simulink model "Demo_3D_Dynamics_cs"  (Simulink 7.6)
settings: Solver=ode5  SolverMode=SingleTasking  StartTime=0.0  StopTime=26  FixedStep=1/200  RelTol=1e-3
model workspace (MAT data in the model file):
  mbox_table.block_array(1).src = 'built-in/Subsystem'
  mbox_table.block_array(1).dest = 'Demo_3D_Dynamics_cs/BMW_X5_1'
  mbox_table.block_array(1).mode = 0
  mbox_table.block_array(2).src = 'simulink/Sinks/Out1'
  mbox_table.block_array(2).dest = 'Demo_3D_Dynamics_cs/BMW_X5_1/STATE_BMW_X5_1'
  mbox_table.block_array(2).mode = 0
  mbox_table.block_array(3).src = 'PreScanSimulinkLibrary/State'
  mbox_table.block_array(3).dest = 'Demo_3D_Dynamics_cs/STATE_BMW_X5_1'
  mbox_table.block_array(3).mode = 0
  mbox_table.block_array(4).src = 'PreScanSimulinkLibrary/PathFollower'
  mbox_table.block_array(4).dest = 'Demo_3D_Dynamics_cs/BMW_X5_1/PathFollower_1'
  mbox_table.block_array(4).mode = 0
  mbox_table.block_array(5).src = 'simulink/Sources/Constant'
  mbox_table.block_array(5).dest = 'Demo_3D_Dynamics_cs/BMW_X5_1/pos'
  mbox_table.block_array(5).mode = 0
  mbox_table.block_array(6).src = 'simulink/Sources/Constant'
  mbox_table.block_array(6).dest = 'Demo_3D_Dynamics_cs/BMW_X5_1/InitialVelocity'
  mbox_table.block_array(6).mode = 0
  mbox_table.block_array(7).src = 'PreScanSimulinkLibrary/Trajectories'
  mbox_table.block_array(7).dest = 'Demo_3D_Dynamics_cs/BMW_X5_1/Trajectories'
  mbox_table.block_array(7).mode = 0
  mbox_table.block_array(8).src = 'simulink/Sources/Constant'
  mbox_table.block_array(8).dest = 'Demo_3D_Dynamics_cs/BMW_X5_1/Trajectories/Trajectory_1_Offset'
  mbox_table.block_array(8).mode = 0
  mbox_table.block_array(9).src = 'PreScanSimulinkLibrary/Trajectory'
  mbox_table.block_array(9).dest = 'Demo_3D_Dynamics_cs/BMW_X5_1/Trajectories/Trajectory_1'
  mbox_table.block_array(9).mode = 0
  mbox_table.block_array(10).src = 'PreScanSimulinkLibrary/Traj2State'
  mbox_table.block_array(10).dest = 'Demo_3D_Dynamics_cs/BMW_X5_1/Trajectories/Traj2State1'
  mbox_table.block_array(10).mode = 0
  mbox_table.block_array(11).src = 'simulink/Sinks/Out1'
  mbox_table.block_array(11).dest = 'Demo_3D_Dynamics_cs/BMW_X5_1/Trajectories/State'
  mbox_table.block_array(11).mode = 0
  mbox_table.block_array(12).src = 'PreScanSimulinkLibrary/SELF'
  mbox_table.block_array(12).dest = 'Demo_3D_Dynamics_cs/SELF_BMW_X5_1'
  mbox_table.block_array(12).mode = 0
  mbox_table.block_array(13).src = 'simulink/Sources/In1'
  mbox_table.block_array(13).dest = 'Demo_3D_Dynamics_cs/BMW_X5_1/SELF_BMW_X5_1'
  mbox_table.block_array(13).mode = 0
  mbox_table.block_array(14).src = 'PreScanSimulinkLibrary/DemuxSELF'
  mbox_table.block_array(14).dest = 'Demo_3D_Dynamics_cs/BMW_X5_1/SELF_Demux'
  mbox_table.block_array(14).mode = 0
  mbox_table.block_array(15).src = 'simulink/Sinks/Out1'
  mbox_table.block_array(15).dest = 'Demo_3D_Dynamics_cs/BMW_X5_1/VISUWheels_BMW_X5_1'
  mbox_table.block_array(15).mode = 0
  mbox_table.block_array(16).src = 'PreScanSimulinkLibrary/VisuWheels'
  mbox_table.block_array(16).dest = 'Demo_3D_Dynamics_cs/VISUWheels_BMW_X5_1'
  mbox_table.block_array(16).mode = 0
  mbox_table.block_array(17).src = 'PreScanSimulinkLibrary/MuxWheels'
  mbox_table.block_array(17).dest = 'Demo_3D_Dynamics_cs/BMW_X5_1/VISUWheels_Mux'
  mbox_table.block_array(17).mode = 0
  mbox_table.block_array(18).src = 'PreScanSimulinkLibrary/Simple_Vehicle_Dynamics_3D'
  mbox_table.block_array(18).dest = 'Demo_3D_Dynamics_cs/BMW_X5_1/Dynamics_Simple_3D'
  mbox_table.block_array(18).mode = 0
  mbox_table.block_array(19).src = 'PreScanSimulinkLibrary/PreScan_Contact_Sensor'
  mbox_table.block_array(19).dest = 'Demo_3D_Dynamics_cs/BMW_X5_1/PreScan_Contact_Sensor'
  mbox_table.block_array(19).mode = 0
  mbox_table.block_array(20).src = 'SimCoreLibrary/SimCoreConfiguration'
  mbox_table.block_array(20).dest = 'Demo_3D_Dynamics_cs/SimCoreConfiguration'
  mbox_table.block_array(20).mode = 0
  mbox_table.block_array(21).src = 'SimCoreLibrary/Actuators'
  mbox_table.block_array(21).dest = 'Demo_3D_Dynamics_cs/Actuators'
  mbox_table.block_array(21).mode = 0
  mbox_table.block_array(22).src = 'SimCoreLibrary/SetActuators'
  mbox_table.block_array(22).dest = 'Demo_3D_Dynamics_cs/SetActuators'
  mbox_table.block_array(22).mode = 0
  mbox_table.block_array(23).src = 'SimCoreLibrary/GetSensors'
  mbox_table.block_array(23).dest = 'Demo_3D_Dynamics_cs/GetSensors'
  mbox_table.block_array(23).mode = 0
  mbox_table.block_array(24).src = 'SimCoreLibrary/SimCoreInfo'
  mbox_table.block_array(24).dest = 'Demo_3D_Dynamics_cs/SimCoreInfo'
  mbox_table.block_array(24).mode = 0
  mbox_table.block_array(25).src = 'PreScanSimulinkLibrary/Regenerate'
  mbox_table.block_array(25).dest = 'Demo_3D_Dynamics_cs/Regenerate'
  mbox_table.block_array(25).mode = 0
  mbox_table.block_array(26).src = 'PreScanSimulinkLibrary/Record for Replay  '
  mbox_table.block_array(26).dest = 'Demo_3D_Dynamics_cs/Record for Replay  '
  mbox_table.block_array(26).mode = 0
  mbox_table.block_array(27).src = 'PreScanSimulinkLibrary/Open Useful Blocks'
  mbox_table.block_array(27).dest = 'Demo_3D_Dynamics_cs/Open Useful Blocks'
  mbox_table.block_array(27).mode = 0
  mbox_table.block_array(28).src = 'PreScanSimulinkLibrary/PreScan Options   '
  mbox_table.block_array(28).dest = 'Demo_3D_Dynamics_cs/PreScan Options   '
  mbox_table.block_array(28).mode = 0
  mbox_table.block_array(29).src = 'built-in/Note'
  mbox_table.block_array(29).dest = 'Demo_3D_Dynamics_cs/Version:                  '
  mbox_table.block_array(29).mode = 0
  mbox_table.block_array(30).src = 'built-in/Note'
  mbox_table.block_array(30).dest = 'Demo_3D_Dynamics_cs/7.4.0'
  mbox_table.block_array(30).mode = 0
  mbox_table.block_array(31).src = 'built-in/Note'
  mbox_table.block_array(31).dest = 'Demo_3D_Dynamics_cs/Author(s):                '
  mbox_table.block_array(31).mode = 0
  mbox_table.block_array(32).src = 'built-in/Note'
  mbox_table.block_array(32).dest = 'Demo_3D_Dynamics_cs/N.A.'
  mbox_table.block_array(32).mode = 0
  mbox_table.block_array(33).src = 'built-in/Note'
  mbox_table.block_array(33).dest = 'Demo_3D_Dynamics_cs/Descriptive text:      '
  mbox_table.block_array(33).mode = 0
  mbox_table.block_array(34).src = 'built-in/Note'
  mbox_table.block_array(34).dest = 'Demo_3D_Dynamics_cs/N.A.'
  mbox_table.block_array(34).mode = 0
  mbox_table.block_array(35).src = 'built-in/Note'
  mbox_table.block_array(35).dest = 'Demo_3D_Dynamics_cs/ID
    | 
    | 18'
  mbox_table.block_array(35).mode = 0
  mbox_table.block_array(36).src = 'built-in/Note'
  mbox_table.block_array(36).dest = 'Demo_3D_Dynamics_cs/OBU-Beacon ID
    | 
    | '
  mbox_table.block_array(36).mode = 0
  mbox_table.block_array(37).src = 'built-in/Note'
  mbox_table.block_array(37).dest = 'Demo_3D_Dynamics_cs/TypeID
    | 
    | 1'
  mbox_table.block_array(37).mode = 0
  mbox_table.block_array(38).src = 'built-in/Note'
  mbox_table.block_array(38).dest = 'Demo_3D_Dynamics_cs/TypeTag
    | 
    | Car'
  mbox_table.block_array(38).mode = 0
  mbox_table.block_array(39).src = 'built-in/Note'
  mbox_table.block_array(39).dest = 'Demo_3D_Dynamics_cs/SD
    | 
    | Y'
  mbox_table.block_array(39).mode = 0
  mbox_table.block_array(40).src = 'built-in/Note'
  mbox_table.block_array(40).dest = 'Demo_3D_Dynamics_cs/CD
    | 
    | N'
  mbox_table.block_array(40).mode = 0
  mbox_table.block_array(41).src = 'built-in/Note'
  mbox_table.block_array(41).dest = 'Demo_3D_Dynamics_cs/Name
    | 
    | BMW_X5_1'
  mbox_table.block_array(41).mode = 0
  mbox_table.block_array(42).src = 'built-in/Note'
  mbox_table.block_array(42).dest = 'Demo_3D_Dynamics_cs/Num ID       OBU-Beacon ID     Type ID      Type Tag             SD        CD             Name                          '
  mbox_table.block_array(42).mode = 0
  mbox_table.block_array(43).src = 'built-in/Ground'
  mbox_table.block_array(43).dest = 'Demo_3D_Dynamics_cs/BMW_X5_1/Ground_1'
  mbox_table.block_array(43).mode = 1
  mbox_table.block_array(44).src = 'built-in/Ground'
  mbox_table.block_array(44).dest = 'Demo_3D_Dynamics_cs/BMW_X5_1/Ground_2'
  mbox_table.block_array(44).mode = 1
  mbox_table.block_array(45).src = 'built-in/Terminator'
  mbox_table.block_array(45).dest = 'Demo_3D_Dynamics_cs/BMW_X5_1/Terminator_1'
  mbox_table.block_array(45).mode = 1
  mbox_table.block_array(46).src = 'built-in/Ground'
  mbox_table.block_array(46).dest = 'Demo_3D_Dynamics_cs/BMW_X5_1/Ground_3'
  mbox_table.block_array(46).mode = 1
  mbox_table.block_array(47).src = 'built-in/Terminator'
  mbox_table.block_array(47).dest = 'Demo_3D_Dynamics_cs/BMW_X5_1/Terminator_2'
  mbox_table.block_array(47).mode = 1
  mbox_table.block_array(48).src = 'built-in/Terminator'
  mbox_table.block_array(48).dest = 'Demo_3D_Dynamics_cs/BMW_X5_1/Terminator_3'
  mbox_table.block_array(48).mode = 1
  mbox_table.block_array(49).src = 'built-in/Ground'
  mbox_table.block_array(49).dest = 'Demo_3D_Dynamics_cs/BMW_X5_1/Ground_4'
  mbox_table.block_array(49).mode = 1
  mbox_table.block_array(50).src = 'built-in/Terminator'
  mbox_table.block_array(50).dest = 'Demo_3D_Dynamics_cs/BMW_X5_1/Terminator_4'
  mbox_table.block_array(50).mode = 1
  mbox_table.block_array(51).src = 'built-in/Terminator'
  mbox_table.block_array(51).dest = 'Demo_3D_Dynamics_cs/BMW_X5_1/Terminator_5'
  mbox_table.block_array(51).mode = 1
  mbox_table.block_array(52).src = 'built-in/Terminator'
  mbox_table.block_array(52).dest = 'Demo_3D_Dynamics_cs/BMW_X5_1/Terminator_6'
  mbox_table.block_array(52).mode = 1
  mbox_table.block_array(53).src = 'built-in/Terminator'
  mbox_table.block_array(53).dest = 'Demo_3D_Dynamics_cs/BMW_X5_1/Terminator_7'
  mbox_table.block_array(53).mode = 1
  mbox_table.block_array(54).src = 'built-in/Terminator'
  mbox_table.block_array(54).dest = 'Demo_3D_Dynamics_cs/BMW_X5_1/Terminator_8'
  mbox_table.block_array(54).mode = 1
  mbox_table.block_array(55).src = 'built-in/Terminator'
  mbox_table.block_array(55).dest = 'Demo_3D_Dynamics_cs/BMW_X5_1/Terminator_9'
  mbox_table.block_array(55).mode = 1
  mbox_table.block_array(56).src = 'built-in/Terminator'
  mbox_table.block_array(56).dest = 'Demo_3D_Dynamics_cs/BMW_X5_1/Terminator_10'
  mbox_table.block_array(56).mode = 1
  mbox_table.block_array(57).src = 'built-in/Terminator'
  mbox_table.block_array(57).dest = 'Demo_3D_Dynamics_cs/BMW_X5_1/Terminator_11'
  mbox_table.block_array(57).mode = 1
  mbox_table.block_array(58).src = 'built-in/Terminator'
  mbox_table.block_array(58).dest = 'Demo_3D_Dynamics_cs/BMW_X5_1/Terminator_12'
  mbox_table.block_array(58).mode = 1
  mbox_table.block_array(59).src = 'built-in/Ground'
  mbox_table.block_array(59).dest = 'Demo_3D_Dynamics_cs/BMW_X5_1/Ground_5'
  mbox_table.block_array(59).mode = 1
  mbox_table.block_index : java.util.Hashtable (value not decoded)
  mbox_table.line_array(1).sys = 'Demo_3D_Dynamics_cs'
  mbox_table.line_array(1).line_id = 'L1'
  mbox_table.line_array(1).iport = 'STATE_BMW_X5_1/1'
  mbox_table.line_array(1).oport = 'BMW_X5_1/1'
  mbox_table.line_array(1).mode = 0
  mbox_table.line_array(2).sys = 'Demo_3D_Dynamics_cs/BMW_X5_1'
  mbox_table.line_array(2).line_id = 'L2'
  mbox_table.line_array(2).iport = 'PathFollower_1/1'
  mbox_table.line_array(2).oport = 'pos/1'
  mbox_table.line_array(2).mode = 0
  mbox_table.line_array(3).sys = 'Demo_3D_Dynamics_cs/BMW_X5_1'
  mbox_table.line_array(3).line_id = 'L3'
  mbox_table.line_array(3).iport = 'PathFollower_1/4'
  mbox_table.line_array(3).oport = 'InitialVelocity/1'
  mbox_table.line_array(3).mode = 0
  mbox_table.line_array(4).sys = 'Demo_3D_Dynamics_cs/BMW_X5_1/Trajectories'
  mbox_table.line_array(4).line_id = 'L4'
  mbox_table.line_array(4).iport = 'Traj2State1/1'
  mbox_table.line_array(4).oport = 'Trajectory_1/1'
  mbox_table.line_array(4).mode = 0
  mbox_table.line_array(5).sys = 'Demo_3D_Dynamics_cs/BMW_X5_1/Trajectories'
  mbox_table.line_array(5).line_id = 'L5'
  mbox_table.line_array(5).iport = 'Traj2State1/2'
  mbox_table.line_array(5).oport = 'Trajectory_1_Offset/1'
  mbox_table.line_array(5).mode = 0
  mbox_table.line_array(6).sys = 'Demo_3D_Dynamics_cs/BMW_X5_1/Trajectories'
  mbox_table.line_array(6).line_id = 'L6'
  mbox_table.line_array(6).iport = 'State/1'
  mbox_table.line_array(6).oport = 'Traj2State1/1'
  mbox_table.line_array(6).mode = 0
  mbox_table.line_array(7).sys = 'Demo_3D_Dynamics_cs'
  mbox_table.line_array(7).line_id = 'L7'
  mbox_table.line_array(7).iport = 'BMW_X5_1/1'
  mbox_table.line_array(7).oport = 'SELF_BMW_X5_1/1'
  mbox_table.line_array(7).mode = 0
  mbox_table.line_array(8).sys = 'Demo_3D_Dynamics_cs/BMW_X5_1'
  mbox_table.line_array(8).line_id = 'L8'
  mbox_table.line_array(8).iport = 'SELF_Demux/1'
  mbox_table.line_array(8).oport = 'SELF_BMW_X5_1/1'
  mbox_table.line_array(8).mode = 0
  mbox_table.line_array(9).sys = 'Demo_3D_Dynamics_cs/BMW_X5_1'
  mbox_table.line_array(9).line_id = 'L9'
  mbox_table.line_array(9).iport = 'VISUWheels_BMW_X5_1/1'
  mbox_table.line_array(9).oport = 'VISUWheels_Mux/1'
  mbox_table.line_array(9).mode = 0
  mbox_table.line_array(10).sys = 'Demo_3D_Dynamics_cs'
  mbox_table.line_array(10).line_id = 'L10'
  mbox_table.line_array(10).iport = 'VISUWheels_BMW_X5_1/1'
  mbox_table.line_array(10).oport = 'BMW_X5_1/2'
  mbox_table.line_array(10).mode = 0
  mbox_table.line_array(11).sys = 'Demo_3D_Dynamics_cs/BMW_X5_1'
  mbox_table.line_array(11).line_id = 'L11'
  mbox_table.line_array(11).iport = 'PreScan_Contact_Sensor/1'
  mbox_table.line_array(11).oport = 'Dynamics_Simple_3D/8'
  mbox_table.line_array(11).mode = 0
  mbox_table.line_array(12).sys = 'Demo_3D_Dynamics_cs/BMW_X5_1'
  mbox_table.line_array(12).line_id = 'L12'
  mbox_table.line_array(12).iport = 'Dynamics_Simple_3D/8'
  mbox_table.line_array(12).oport = 'PreScan_Contact_Sensor/1'
  mbox_table.line_array(12).mode = 0
  mbox_table.line_array(13).sys = 'Demo_3D_Dynamics_cs/BMW_X5_1'
  mbox_table.line_array(13).line_id = 'L13'
  mbox_table.line_array(13).iport = 'VISUWheels_Mux/3'
  mbox_table.line_array(13).oport = 'Dynamics_Simple_3D/2'
  mbox_table.line_array(13).mode = 0
  mbox_table.line_array(14).sys = 'Demo_3D_Dynamics_cs/BMW_X5_1'
  mbox_table.line_array(14).line_id = 'L14'
  mbox_table.line_array(14).iport = 'VISUWheels_Mux/4'
  mbox_table.line_array(14).oport = 'Dynamics_Simple_3D/4'
  mbox_table.line_array(14).mode = 0
  mbox_table.line_array(15).sys = 'Demo_3D_Dynamics_cs/BMW_X5_1'
  mbox_table.line_array(15).line_id = 'L15'
  mbox_table.line_array(15).iport = 'VISUWheels_Mux/5'
  mbox_table.line_array(15).oport = 'Dynamics_Simple_3D/5'
  mbox_table.line_array(15).mode = 0
  mbox_table.line_array(16).sys = 'Demo_3D_Dynamics_cs/BMW_X5_1'
  mbox_table.line_array(16).line_id = 'L16'
  mbox_table.line_array(16).iport = 'VISUWheels_Mux/6'
  mbox_table.line_array(16).oport = 'Dynamics_Simple_3D/6'
  mbox_table.line_array(16).mode = 0
  mbox_table.line_array(17).sys = 'Demo_3D_Dynamics_cs/BMW_X5_1'
  mbox_table.line_array(17).line_id = 'L17'
  mbox_table.line_array(17).iport = 'VISUWheels_Mux/7'
  mbox_table.line_array(17).oport = 'Dynamics_Simple_3D/7'
  mbox_table.line_array(17).mode = 0
  mbox_table.line_array(18).sys = 'Demo_3D_Dynamics_cs/BMW_X5_1'
  mbox_table.line_array(18).line_id = 'L18'
  mbox_table.line_array(18).iport = 'Dynamics_Simple_3D/1'
  mbox_table.line_array(18).oport = 'PathFollower_1/1'
  mbox_table.line_array(18).mode = 0
  mbox_table.line_array(19).sys = 'Demo_3D_Dynamics_cs/BMW_X5_1'
  mbox_table.line_array(19).line_id = 'L19'
  mbox_table.line_array(19).iport = 'Dynamics_Simple_3D/2'
  mbox_table.line_array(19).oport = 'PathFollower_1/2'
  mbox_table.line_array(19).mode = 0
  mbox_table.line_array(20).sys = 'Demo_3D_Dynamics_cs/BMW_X5_1'
  mbox_table.line_array(20).line_id = 'L20'
  mbox_table.line_array(20).iport = 'Dynamics_Simple_3D/3'
  mbox_table.line_array(20).oport = 'PathFollower_1/3'
  mbox_table.line_array(20).mode = 0
  mbox_table.line_array(21).sys = 'Demo_3D_Dynamics_cs/BMW_X5_1'
  mbox_table.line_array(21).line_id = 'L21'
  mbox_table.line_array(21).iport = 'Dynamics_Simple_3D/4'
  mbox_table.line_array(21).oport = 'PathFollower_1/4'
  mbox_table.line_array(21).mode = 0
  mbox_table.line_array(22).sys = 'Demo_3D_Dynamics_cs/BMW_X5_1'
  mbox_table.line_array(22).line_id = 'L22'
  mbox_table.line_array(22).iport = 'Dynamics_Simple_3D/6'
  mbox_table.line_array(22).oport = 'PathFollower_1/5'
  mbox_table.line_array(22).mode = 0
  mbox_table.line_array(23).sys = 'Demo_3D_Dynamics_cs/BMW_X5_1'
  mbox_table.line_array(23).line_id = 'L23'
  mbox_table.line_array(23).iport = 'PathFollower_1/6'
  mbox_table.line_array(23).oport = 'SELF_Demux/10'
  mbox_table.line_array(23).mode = 0
  mbox_table.line_array(24).sys = 'Demo_3D_Dynamics_cs/BMW_X5_1'
  mbox_table.line_array(24).line_id = 'L24'
  mbox_table.line_array(24).iport = 'STATE_BMW_X5_1/1'
  mbox_table.line_array(24).oport = 'Dynamics_Simple_3D/1'
  mbox_table.line_array(24).mode = 0
  mbox_table.line_array(25).sys = 'Demo_3D_Dynamics_cs/BMW_X5_1'
  mbox_table.line_array(25).line_id = 'l1'
  mbox_table.line_array(25).iport = 'Dynamics_Simple_3D/5'
  mbox_table.line_array(25).oport = 'Ground_1/1'
  mbox_table.line_array(25).mode = 1
  mbox_table.line_array(26).sys = 'Demo_3D_Dynamics_cs/BMW_X5_1'
  mbox_table.line_array(26).line_id = 'l2'
  mbox_table.line_array(26).iport = 'Dynamics_Simple_3D/7'
  mbox_table.line_array(26).oport = 'Ground_2/1'
  mbox_table.line_array(26).mode = 1
  mbox_table.line_array(27).sys = 'Demo_3D_Dynamics_cs/BMW_X5_1'
  mbox_table.line_array(27).line_id = 'l3'
  mbox_table.line_array(27).iport = 'Terminator_1/1'
  mbox_table.line_array(27).oport = 'Dynamics_Simple_3D/3'
  mbox_table.line_array(27).mode = 1
  mbox_table.line_array(28).sys = 'Demo_3D_Dynamics_cs/BMW_X5_1'
  mbox_table.line_array(28).line_id = 'l4'
  mbox_table.line_array(28).iport = 'PathFollower_1/2'
  mbox_table.line_array(28).oport = 'Ground_3/1'
  mbox_table.line_array(28).mode = 1
  mbox_table.line_array(29).sys = 'Demo_3D_Dynamics_cs/BMW_X5_1'
  mbox_table.line_array(29).line_id = 'l5'
  mbox_table.line_array(29).iport = 'Terminator_2/1'
  mbox_table.line_array(29).oport = 'PathFollower_1/6'
  mbox_table.line_array(29).mode = 1
  mbox_table.line_array(30).sys = 'Demo_3D_Dynamics_cs/BMW_X5_1'
  mbox_table.line_array(30).line_id = 'l6'
  mbox_table.line_array(30).iport = 'Terminator_3/1'
  mbox_table.line_array(30).oport = 'PathFollower_1/7'
  mbox_table.line_array(30).mode = 1
  mbox_table.line_array(31).sys = 'Demo_3D_Dynamics_cs/BMW_X5_1'
  mbox_table.line_array(31).line_id = 'l7'
  mbox_table.line_array(31).iport = 'PreScan_Contact_Sensor/3'
  mbox_table.line_array(31).oport = 'Ground_4/1'
  mbox_table.line_array(31).mode = 1
  mbox_table.line_array(32).sys = 'Demo_3D_Dynamics_cs/BMW_X5_1'
  mbox_table.line_array(32).line_id = 'l8'
  mbox_table.line_array(32).iport = 'Terminator_4/1'
  mbox_table.line_array(32).oport = 'SELF_Demux/3'
  mbox_table.line_array(32).mode = 1
  mbox_table.line_array(33).sys = 'Demo_3D_Dynamics_cs/BMW_X5_1'
  mbox_table.line_array(33).line_id = 'l9'
  mbox_table.line_array(33).iport = 'Terminator_5/1'
  mbox_table.line_array(33).oport = 'SELF_Demux/4'
  mbox_table.line_array(33).mode = 1
  mbox_table.line_array(34).sys = 'Demo_3D_Dynamics_cs/BMW_X5_1'
  mbox_table.line_array(34).line_id = 'l10'
  mbox_table.line_array(34).iport = 'Terminator_6/1'
  mbox_table.line_array(34).oport = 'SELF_Demux/5'
  mbox_table.line_array(34).mode = 1
  mbox_table.line_array(35).sys = 'Demo_3D_Dynamics_cs/BMW_X5_1'
  mbox_table.line_array(35).line_id = 'l11'
  mbox_table.line_array(35).iport = 'Terminator_7/1'
  mbox_table.line_array(35).oport = 'SELF_Demux/7'
  mbox_table.line_array(35).mode = 1
  mbox_table.line_array(36).sys = 'Demo_3D_Dynamics_cs/BMW_X5_1'
  mbox_table.line_array(36).line_id = 'l12'
  mbox_table.line_array(36).iport = 'Terminator_8/1'
  mbox_table.line_array(36).oport = 'SELF_Demux/8'
  mbox_table.line_array(36).mode = 1
  mbox_table.line_array(37).sys = 'Demo_3D_Dynamics_cs/BMW_X5_1'
  mbox_table.line_array(37).line_id = 'l13'
  mbox_table.line_array(37).iport = 'Terminator_9/1'
  mbox_table.line_array(37).oport = 'SELF_Demux/9'
  mbox_table.line_array(37).mode = 1
  mbox_table.line_array(38).sys = 'Demo_3D_Dynamics_cs/BMW_X5_1'
  mbox_table.line_array(38).line_id = 'l14'
  mbox_table.line_array(38).iport = 'Terminator_10/1'
  mbox_table.line_array(38).oport = 'SELF_Demux/11'
  mbox_table.line_array(38).mode = 1
  mbox_table.line_array(39).sys = 'Demo_3D_Dynamics_cs/BMW_X5_1'
  mbox_table.line_array(39).line_id = 'l15'
  mbox_table.line_array(39).iport = 'Terminator_11/1'
  mbox_table.line_array(39).oport = 'SELF_Demux/12'
  mbox_table.line_array(39).mode = 1
  mbox_table.line_array(40).sys = 'Demo_3D_Dynamics_cs/BMW_X5_1'
  mbox_table.line_array(40).line_id = 'l16'
  mbox_table.line_array(40).iport = 'Terminator_12/1'
  mbox_table.line_array(40).oport = 'Trajectories/1'
  mbox_table.line_array(40).mode = 1
  mbox_table.line_array(41).sys = 'Demo_3D_Dynamics_cs/BMW_X5_1'
  mbox_table.line_array(41).line_id = 'l17'
  mbox_table.line_array(41).iport = 'VISUWheels_Mux/2'
  mbox_table.line_array(41).oport = 'Ground_5/1'
  mbox_table.line_array(41).mode = 1
  mbox_table.line_index : java.util.Hashtable (value not decoded)
  mbox_table.next_linenr = 25
  mbox_table.next_termlinenr = 18
  model_closed = 0
  sim_status = 0
PreLoadFcn:
  | check_NUTS_defined;
  | 
  | assignin('base',['model_closed_' bdroot],false);
InitFcn:
  | PreScanExperimentInitFcn(bdroot)
StopFcn:
  | PreScanExperimentStopFcn(bdroot)
undefined symbols (not defined in the file): DiscIntNeverNeededParam, x_ini_VRML, y_ini_VRML, z_ini_VRML
libraries: simulink x37, simulink_extras x11, PreScanSimulinkLibrary x10, simulink_need_slupdate x1, PreScanUsefulBlocks x1
(part 1 of 5)
CloseFcn:
  | evalin('base',['clear model_closed_' bdroot]);
settings Model: Creator=PRESCAN  LastModifiedBy=buildbot
settings OptimizationCC: InitFltsAndDblsToZero=on
settings DebuggingCC: SaveWithParameterizedLinksMsg=none  SignalResolutionControl=TryResolveAllWithWarning  SolverPrmCheckMsg=none  MultiTaskDSMMsg=warning  MultiTaskCondExecSysMsg=none
settings RTWCC: IncludeERTFirstTime=on
settings GRTTargetCC: TargetFcnLib=ansi_tfl_tmw.mat

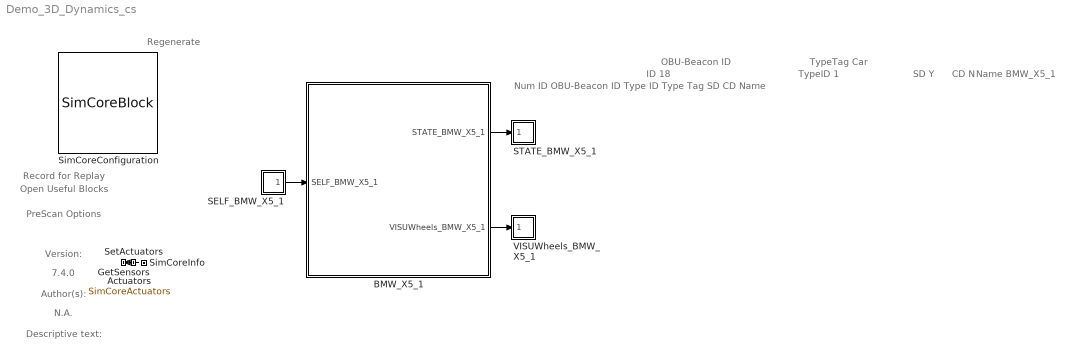
== system Demo_3D_Dynamics_cs ==
  note: Regenerate
  note: Record for Replay
  note: Open Useful Blocks
  note: PreScan Options
  note: Version:
  note: 7.4.0
  note: Author(s):
  note: N.A.
  note: Descriptive text:
  note: ID
      |
      | 18
  note: OBU-Beacon ID
  note: TypeID
      |
      | 1
  note: TypeTag
      |
      | Car
  note: SD
      |
      | Y
  note: CD
      |
      | N
  note: Name
      |
      | BMW_X5_1
  note: Num ID OBU-Beacon ID Type ID Type Tag SD CD Name
  Actuators : DataStoreMemory  Tag=Actuators  DataStoreName=SimCoreActuators  InitialValue=zeros(43,1)
      settings: DeleteFcn=PreScanBlockDeleteFcn;
  BMW_X5_1 : Subsystem  Tag=WorldObjectSubSystem  InitFcn=UniqueId = '276';
      mask Display: image(imread('BMW_X5.jpg'));color('white');text(0,0,' ID=18\n')
  GetSensors : Subsystem  Tag=GetSensors  Priority=2  mask(PreScan Simulation Core Block){NrOfSensors=8, TimeStep=10/200}
      mask prompts: NrOfSensors "Number of sensor values"; TimeStep "Timestep [s]"
      mask help:
      | Please do not remove this block from the PreScan compilation sheet,
      | as it contains essential configuration parameters for a PreScan simulation.
      settings: DeleteFcn=PreScanBlockDeleteFcn;
  SELF_BMW_X5_1 : Subsystem  Tag=SELF  Priority=3  mask(PreScan Source Block: SELF){PortName=SELF_BMW_X5_1, PortIndex=0, PortWidth=8, TimeStep=10/200}
      mask prompts: PortName "Auto-Assigned: Port Name [-]"; PortIndex "Auto-Assigned: Port Index [-]"; PortWidth "Auto-Assigned: Port Dimensions"; TimeStep "Auto-Assigned: Upload Period [s]"
      mask help:
      | The SELF port shows (state) information of the actor itself. The outputs are position in the experiment's axis system and the GPS coordinates, and the object's absolute velocity and compass heading.
      |
      | For more information, please click Help.
      settings: DeleteFcn=PreScanBlockDeleteFcn;
      mask Help: eval('openHelp(462)')
      mask Display: image(imread('GPS.png'))
  STATE_BMW_X5_1 : Subsystem  Tag=State  Priority=0  mask(PreScan Sink Block: State){x0=40, y0=28.25, z0=0.69, Roll0=0, Pitch0=0, Yaw0=0, TimeStep=10/200}
      mask prompts: x0 "Ini x-position VEHICLE wrt GLOBAL axis system [m]"; y0 "Ini y-position VEHICLE wrt GLOBAL axis system [m]"; z0 "Ini z-position VEHICLE wrt GLOBAL axis system [m]"; Roll0 "Ini roll-angle BODY wrt VEHICLE axis system [deg]"; Pitch0 "Ini pitch-angle BODY wrt VEHICLE axis system [deg]"; Yaw0 "Ini yaw-angle VEHICLE wrt GLOBAL axis system [deg]"; TimeStep "Time Step [s]"
      mask help:
      | The Actor State contains a vector signal of size (9x1), containing the following signals:
      |
      | -  Position                  (x,y,z)                                     [m]
      | -  Velocity                  (vx,vy,vz)                               [m/s]
      | -  Angles                    (Roll, Pitch, Yaw)                   [rad]
      |
      | The Actor state is defined in the global axis system.
      | The state is superponed on the Initial position defined in the GUI.
      |
      | For more information, please click Help.
      settings: DeleteFcn=PreScanBlockDeleteFcn;
      mask Help: eval('openHelp(222)')
      mask Display: image(imread('State.png'))
  SetActuators : Subsystem  Tag=SetActuators  Priority=1  mask(PreScan Simulation Core Block){TimeStep=10/200, NrOfActuators=43}
      mask prompts: TimeStep "Timestep [s]"; NrOfActuators "Number of actuator values"
      mask help:
      | Please do not remove this block from the PreScan compilation sheet,
      | as it contains essential configuration parameters for a PreScan simulation.
      settings: DeleteFcn=PreScanBlockDeleteFcn;
  SimCoreConfiguration : M-S-Function  Tag=SimCoreConfiguration  Description=2F8DE11AFA9E2D1E60DFF0BB6A25510BB705AF952DBBD0EADC2C0AF755B6A15B  FunctionName=SimCoreBlock  Parameters=ExperimentXML PortsXML SimulationCore HostName CheckStart EnableLog RfR EnableGPUAccel ShowComputationTime  mask(PreScan Simulation Core Configurator){SimulationCore=NUTS, HostName=0, CheckStart=0, prescanversion='7.4.0', EnableLog=off, RfR=0, EnableGPUAccel=off, ShowComputationTime=off}
      mask prompts: SimulationCore "Simulation Core"; HostName "Simulation Host"; CheckStart "Show START Dialog"; prescanversion "PreScan Version"; EnableLog "Create TA Log"; RfR "Record for Replay"; EnableGPUAccel "Enable GPU Acceleration"; ShowComputationTime "Show ComputationTime Scope"
      mask help:
      | Please do not remove this block from the PreScan compilation sheet,
      | as it contains essential configuration parameter for a PreScan simulation.
      mask init:
      | model = bdroot;
      | ExperimentXML = [model(1:end-3) '.pex'];
      | PortsXML = [model '_ports.pcd'];
      settings: DeleteFcn=PreScanBlockDeleteFcn;  ModelCloseFcn=assignin('base',['model_closed_' bdroot],true);
      mask Help: eval('openHelp(812)')
      mask Display: image(imread('prescanlogo.ico'))
  SimCoreInfo : Subsystem  Tag=SimCoreInfo
  VISUWheels_BMW_X5_1 : Subsystem  Tag=VisuWheels  Priority=0
      settings: DeleteFcn=PreScanBlockDeleteFcn;
      mask Type: PreScan Sink Block: VisuWheels
      mask Description:
      | The VisuWheels block provides a way to animate the wheels of a vehicle, with steering, rotation (because of velocity) and z-displacement.
      | 
      | For more information, please click Help.
      mask Help: eval('openHelp(223)')
      mask Display: image(imread('wheel.png'))
  wires:
  BMW_X5_1/1(STATE_BMW_X5_1) -> STATE_BMW_X5_1/1(State)
  SELF_BMW_X5_1/1(U) -> BMW_X5_1/1(SELF_BMW_X5_1)
  BMW_X5_1/2(VISUWheels_BMW_X5_1) -> VISUWheels_BMW_X5_1/1(Wheels)
  SetActuators/1(dummy) -> GetSensors/1(dummy)

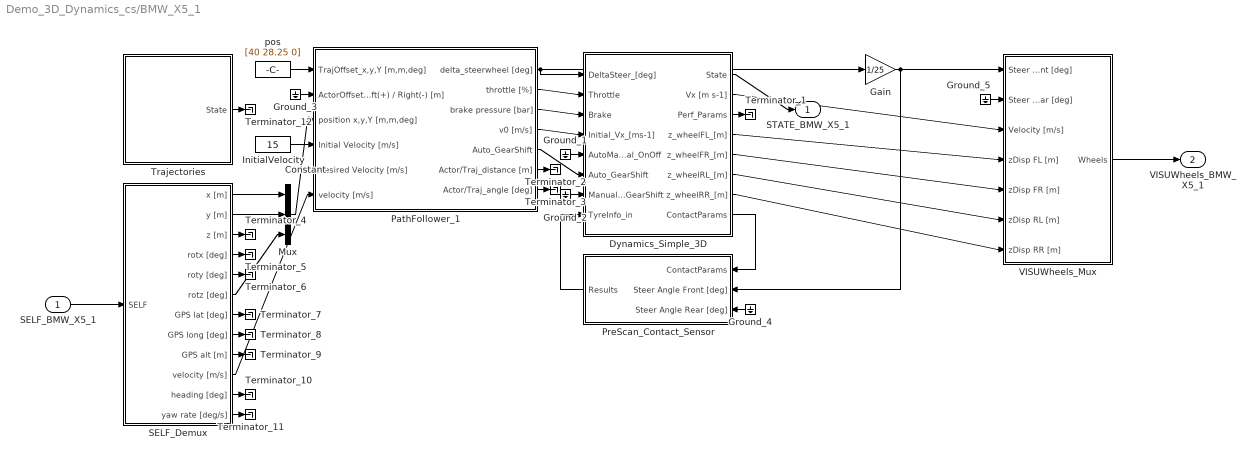
== system Demo_3D_Dynamics_cs/BMW_X5_1 ==
  SELF_BMW_X5_1 : Inport  Tag=SELFInport
  Constant : Constant  Value=15
  Dynamics_Simple_3D : Subsystem  Tag=Simple_Vehicle_Dynamics_3D  mask(PreScan Block: Simple Dynamics 3D){Migrate=on, TimeStep=1/200, ComputationMode=Continuous_Time}
      mask prompts: Migrate "Migrate. During migration this block will be replaced by a newer one."; TimeStep "Auto assigned: Time Step [s]"; ComputationMode "Computation mode:"
      mask help:
      | The Simple Dynamics Model is selected in the GUI to simulate vehicle dynamics behavior.
      |
      | The Simple Dynamics Model is completely open to the user. The parameters of this model can be set in the Simple Dynamics dialog in the GUI.
      |
      | For more information, please click Help.
      mask init:
      | p = SimpleDyn_pars;
      settings: DeleteFcn=PreScanBlockDeleteFcn;
      mask Help: eval('openHelp(234)')
      mask Display:
      | image(imread('SimpleDyn.png'))
      | port_label('input', 1, '{\delta}_S_t_ _e_e_r [deg]','texmode','on')
      | port_label('input', 2, 'Throttle [%]')
      | port_label('input', 3, 'Brake Pres [bar]')
      | port_label('input', 4, 'V_0 [ms-1]','texmode','on')
      | port_label('input', 5, 'Auto=[0]/Manual=[1]')
      | port_label('input', 6, 'Auto_GearShift')
      | port_label('input', 7, 'Manual_GearShift')
      | port_label('input', 8, 'TyreInfo_in')
      | port_label('output', 1, 'State')
      | port_label('output', 2, 'Vx [ms-1]')
      | port_label('output', 3, 'Perf Params')
      | port_label('output', 4, 'zDispFL[m]')
      | port_label('output', 5, 'zDispFR[m]')
      | port_label('output', 6, 'zDispRL[m]')
      | port_label('output', 7, 'zDispRR[m]')
  Gain : Gain  Gain=1/25
  Ground_{1..5} (5 alike) : Ground
  InitialVelocity : Constant  Tag=InitialVelocity  Value=15
  Mux : Mux  Inputs=3
  PathFollower_1 : Subsystem  Tag=pathFollower  mask(PreScan Block: Path Follower){Migrate=on, FileName='Trajectory_1.mat', TunableSteeringGain=1, XShifting_wrt_COG=0}
      mask prompts: Migrate "Migrate. During migration this block will be replaced by a newer one."; FileName "Trajectory Name"; TunableSteeringGain "TunableSteeringGain [-]"; XShifting_wrt_COG "XShifting_wrt_COG [m]"
      mask help:
      | The Path Follower Model is selected in the GUI to simulate driver behavior.
      |
      | For more information, please click Help.
      mask init:
      | load(['trajectories/',eval(FileName)])
      | traject=trajectory';
      | 
      | Traj_x=traject(:,2);
      | Traj_y=traject(:,3);
      | Traj_z=traject(:,4);
      | Traj_vx=traject(:,8);
      | Traj_vy=traject(:,9);
      | Traj_vz=traject(:,10);
      mask Help: eval('openHelp(232)')
  PreScan_Contact_Sensor : Subsystem  Tag=PreScan_Contact_Sensor  mask(PreScan Block: PreScan Contact Sensor){x0=40, y0=28.25, z0=0.69, Roll0=0, Pitch0=0, Yaw0=0, wheelRadius=0.37, hcog=0.69, b=1.69, TimeStep=1/200}
      mask prompts: x0 "Ini x-position VEHICLE wrt GLOBAL axis system [m]"; y0 "Ini y-position VEHICLE wrt GLOBAL axis system [m]"; z0 "Ini z-position VEHICLE wrt GLOBAL axis system [m]"; Roll0 "Ini roll-angle BODY wrt VEHICLE axis system [deg]"; Pitch0 "Ini pitch-angle BODY wrt VEHICLE axis system [deg]"; Yaw0 "Ini yaw-angle VEHICLE wrt GLOBAL axis system [deg]"; wheelRadius "Wheel Radius [m]"; hcog "Dynamics: hCoG [m]"; b "Dynamics: b [m]"; TimeStep "Time Step [s]"
      mask help:
      | This block encapsulates the base Contact sensor.
      |
      | It takes input parameters from the PreScan 3D vehicle dynamics block and outputs contact results.
      mask Help: eval('openHelp(251)')
  SELF_Demux : Subsystem  Tag=DemuxSELF
      settings: DeleteFcn=PreScanBlockDeleteFcn;
      mask Type: PreScan Demux Block:
      mask Display:
      | port_label('output',1,'x [m]')
      | port_label('output',2,'y [m]')
      | port_label('output',3,'z [m]','texmode','on')
      | port_label('output',4,'Rotx [deg]','texmode','on')
      | port_label('output',5,'Roty [deg]','texmode','on')
      | port_label('output',6,'Rotz [deg]','texmode','on')
      | port_label('output',7,'GPS lat [deg]','texmode','on')
      | port_label('output',8,'GPS long [deg]','texmode','on')
      | port_label('output',9,'GPS alt [m]','texmode','on')
      | port_label('output',10,'Velocity [m/s]')
      | port_label('output',11,'Heading [deg]')
      | port_label('output',12,'Yaw rate [deg/s]')
  Terminator_{1..12} (12 alike) : Terminator
  Trajectories : Subsystem  Tag=Trajectories
      settings: DeleteFcn=PreScanBlockDeleteFcn;
      mask Type: PreScan Source Block: Trajectories
      mask Description:
      | The Trajectory block contains the trajectories defined in the PreScan Experiment Editor. The output of the trajectory block is the (vehicle) State.
      | 
      | For more information, please click Help.
      mask Help: eval('openHelp(312)')
      mask Display: image(imread('Trajectory.png'));
  VISUWheels_Mux : Subsystem  Tag=MuxWheels  mask(PreScan Mux Block:){TimeStep=10/200}
      mask prompts: TimeStep "Auto Assigned: Time Step [s]"
      settings: DeleteFcn=PreScanBlockDeleteFcn;
  pos : Constant  Tag=pos  Value=[40 28.25 0]
  STATE_BMW_X5_1 : Outport  Tag=StateOutport
  VISUWheels_BMW_X5_1 : Outport  Tag=VisuWheelsOutport  Port=2  SampleTime=10/200
  wires:
  pos/1 -> PathFollower_1/1(TrajOffset_x,y,Y [m,m,deg])
  InitialVelocity/1 -> PathFollower_1/4(Initial Velocity [m/s])
  SELF_BMW_X5_1/1 -> SELF_Demux/1(SELF)
  VISUWheels_Mux/1(Wheels) -> VISUWheels_BMW_X5_1/1
  Dynamics_Simple_3D/8(ContactParams) -> PreScan_Contact_Sensor/1(ContactParams)
  PreScan_Contact_Sensor/1(Results) -> Dynamics_Simple_3D/8(TyreInfo_in)
  Dynamics_Simple_3D/2(Vx [m s-1]) -> VISUWheels_Mux/3(Velocity [m/s])
  Dynamics_Simple_3D/4(z_wheelFL_[m]) -> VISUWheels_Mux/4(zDisp FL [m])
  Dynamics_Simple_3D/5(z_wheelFR_[m]) -> VISUWheels_Mux/5(zDisp FR [m])
  Dynamics_Simple_3D/6(z_wheelRL_[m]) -> VISUWheels_Mux/6(zDisp RL [m])
  Dynamics_Simple_3D/7(z_wheelRR_[m]) -> VISUWheels_Mux/7(zDisp RR [m])
  PathFollower_1/1(delta_steerwheel [deg]) -> Dynamics_Simple_3D/1(DeltaSteer_[deg]), Gain/1
  PathFollower_1/2(throttle [%]) -> Dynamics_Simple_3D/2(Throttle)
  PathFollower_1/3(brake pressure [bar]) -> Dynamics_Simple_3D/3(Brake)
  PathFollower_1/4(v0 [m/s]) -> Dynamics_Simple_3D/4(Initial_Vx_[ms-1])
  PathFollower_1/5(Auto_GearShift) -> Dynamics_Simple_3D/6(Auto_GearShift)
  Dynamics_Simple_3D/1(State) -> STATE_BMW_X5_1/1
  Gain/1 -> VISUWheels_Mux/1(Steer Angle Front [deg]), PreScan_Contact_Sensor/2(Steer Angle Front [deg])
  SELF_Demux/10(velocity [m/s]) -> PathFollower_1/6(velocity [m/s])
  Mux/1 -> PathFollower_1/3(position x,y,Y [m,m,deg])
  SELF_Demux/6(rotz [deg]) -> Mux/3
  Constant/1 -> PathFollower_1/5(Desired Velocity [m/s])
  SELF_Demux/2(y [m]) -> Mux/2
  SELF_Demux/1(x [m]) -> Mux/1
  Ground_1/1 -> Dynamics_Simple_3D/5(AutoManual_OnOff)
  Ground_2/1 -> Dynamics_Simple_3D/7(Manual_GearShift)
  Dynamics_Simple_3D/3(Perf_Params) -> Terminator_1/1
  Ground_3/1 -> PathFollower_1/2(ActorOffset_Left(+) / Right(-) [m])
  PathFollower_1/6(Actor/Traj_distance [m]) -> Terminator_2/1
  PathFollower_1/7(Actor/Traj_angle [deg]) -> Terminator_3/1
  Ground_4/1 -> PreScan_Contact_Sensor/3(Steer Angle Rear [deg])
  SELF_Demux/3(z [m]) -> Terminator_4/1
  SELF_Demux/4(rotx [deg]) -> Terminator_5/1
  SELF_Demux/5(roty [deg]) -> Terminator_6/1
  SELF_Demux/7(GPS lat [deg]) -> Terminator_7/1
  SELF_Demux/8(GPS long [deg]) -> Terminator_8/1
  SELF_Demux/9(GPS alt [m]) -> Terminator_9/1
  SELF_Demux/11(heading [deg]) -> Terminator_10/1
  SELF_Demux/12(yaw rate [deg/s]) -> Terminator_11/1
  Trajectories/1(State) -> Terminator_12/1
  Ground_5/1 -> VISUWheels_Mux/2(Steer Angle Rear [deg])

== system Demo_3D_Dynamics_cs/GetSensors ==
  dummy : Inport
  GetSensors : M-S-Function  FunctionName=GetSensorsBlock  Parameters=TimeStep NrOfSensors
  tag scope: SimCoreSensors=global
  wires:
  GetSensors/1 -> [SimCoreSensors]
  dummy/1 -> GetSensors/1

== system Demo_3D_Dynamics_cs/SELF_BMW_X5_1 ==
  Selector : Selector  IndexMode=Zero-based  IndexOptions=Starting index (dialog)  Indices=PortIndex  OutputSizes=PortWidth(1)
  U : Outport
  wires:
  Selector/1 -> U/1
  [SimCoreSensors] -> Selector/1

== system Demo_3D_Dynamics_cs/STATE_BMW_X5_1 ==
  State : Inport  SampleTime=TimeStep
  Acceleration : Subsystem  mask(ToSensorWorld){PortName=Acceleration_BMW_X5_1, PortIndex=6, PortWidth=3, TimeStep=10/200}
      mask prompts: PortName "Port Name [-]"; PortIndex "Index [-]"; PortWidth "Port Dimensions [-]"; TimeStep "Upload Period [s]"
      mask help: Sends signal(s) from Simulink to the Sensor World
      mask Help:
      | Sends signal(s) from Simulink to the Sensor World.
      | 
      | - Port Name [-]: specifies the name of the output terminal of the Simulink block.
      | - Index [-]: specifies the start position in the output vector sent to the Sensor World
      | - Port dimensions [-]: specifies the width (number of scalars) of the output port
      | - Upload period [s]: specifies the upload period (in seconds) of the port.
      mask Display: port_label('input', 1, PortName)
  Demux : Demux  Outputs=5
  Position : Subsystem  mask(ToSensorWorld){PortName=Position_BMW_X5_1, PortIndex=0, PortWidth=3, TimeStep=10/200}
      mask prompts: PortName "Port Name [-]"; PortIndex "Index [-]"; PortWidth "Port Dimensions [-]"; TimeStep "Upload Period [s]"
      mask help: Sends signal(s) from Simulink to the Sensor World
      mask Help:
      | Sends signal(s) from Simulink to the Sensor World.
      | 
      | - Port Name [-]: specifies the name of the output terminal of the Simulink block.
      | - Index [-]: specifies the start position in the output vector sent to the Sensor World
      | - Port dimensions [-]: specifies the width (number of scalars) of the output port
      | - Upload period [s]: specifies the upload period (in seconds) of the port.
      mask Display: port_label('input', 1, PortName)
  RPY : Subsystem  mask(ToSensorWorld){PortName=RPY_BMW_X5_1, PortIndex=9, PortWidth=3, TimeStep=10/200}
      mask prompts: PortName "Port Name [-]"; PortIndex "Index [-]"; PortWidth "Port Dimensions [-]"; TimeStep "Upload Period [s]"
      mask help: Sends signal(s) from Simulink to the Sensor World
      mask Help:
      | Sends signal(s) from Simulink to the Sensor World.
      | 
      | - Port Name [-]: specifies the name of the output terminal of the Simulink block.
      | - Index [-]: specifies the start position in the output vector sent to the Sensor World
      | - Port dimensions [-]: specifies the width (number of scalars) of the output port
      | - Upload period [s]: specifies the upload period (in seconds) of the port.
      mask Display: port_label('input', 1, PortName)
  Velocity : Subsystem  mask(ToSensorWorld){PortName=Velocity_BMW_X5_1, PortIndex=3, PortWidth=3, TimeStep=10/200}
      mask prompts: PortName "Port Name [-]"; PortIndex "Index [-]"; PortWidth "Port Dimensions [-]"; TimeStep "Upload Period [s]"
      mask help: Sends signal(s) from Simulink to the Sensor World
      mask Help:
      | Sends signal(s) from Simulink to the Sensor World.
      | 
      | - Port Name [-]: specifies the name of the output terminal of the Simulink block.
      | - Index [-]: specifies the start position in the output vector sent to the Sensor World
      | - Port dimensions [-]: specifies the width (number of scalars) of the output port
      | - Upload period [s]: specifies the upload period (in seconds) of the port.
      mask Display: port_label('input', 1, PortName)
  iniBODYAngles wrtVEH [rad] : Constant  Value=[Roll0 Pitch0 0]  SampleTime=TimeStep
  iniVEHAngles wrtGLOB [rad] : Constant  Value=[0 0 Yaw0]  SampleTime=TimeStep
  iniVEHposition wrtGLOB [m] : Constant  Value=[x0 y0 z0]  SampleTime=TimeStep
  state2FullState : PreScanSimulinkLibrary/state2FullState  SystemSampleTime=-1
  velRPY : Subsystem  mask(ToSensorWorld){PortName=velRPY_BMW_X5_1, PortIndex=12, PortWidth=3, TimeStep=10/200}
      mask prompts: PortName "Port Name [-]"; PortIndex "Index [-]"; PortWidth "Port Dimensions [-]"; TimeStep "Upload Period [s]"
      mask help: Sends signal(s) from Simulink to the Sensor World
      mask Help:
      | Sends signal(s) from Simulink to the Sensor World.
      | 
      | - Port Name [-]: specifies the name of the output terminal of the Simulink block.
      | - Index [-]: specifies the start position in the output vector sent to the Sensor World
      | - Port dimensions [-]: specifies the width (number of scalars) of the output port
      | - Upload period [s]: specifies the upload period (in seconds) of the port.
      mask Display: port_label('input', 1, PortName)
  wires:
  Demux/5 -> velRPY/1(Y)
  Demux/4 -> RPY/1(Y)
  Demux/3 -> Acceleration/1(Y)
  Demux/2 -> Velocity/1(Y)
  Demux/1 -> Position/1(Y)
  State/1 -> state2FullState/1
  state2FullState/1 -> Demux/1
  iniVEHposition wrtGLOB [m]/1 -> state2FullState/2
  iniBODYAngles wrtVEH [rad]/1 -> state2FullState/3
  iniVEHAngles wrtGLOB [rad]/1 -> state2FullState/4

== system Demo_3D_Dynamics_cs/SetActuators ==
  Bus Creator : BusCreator  Inputs=1
  Data Store Read : DataStoreRead  DataStoreName=SimCoreActuators  SampleTime=TimeStep
  SendActuators : M-S-Function  FunctionName=SendActuatorsBlock  Parameters=TimeStep NrOfActuators
  dummy : Outport
  tag scope: SimCoreInfo=global
  wires:
  Bus Creator/1 -> [SimCoreInfo]  "SimCore"
  SendActuators/2 -> Bus Creator/1  "ComputationTime[s]"
  SendActuators/1 -> dummy/1
  Data Store Read/1 -> SendActuators/1

== system Demo_3D_Dynamics_cs/SimCoreInfo ==
  Bus Selector : BusSelector  OutputSignals=ComputationTime[s]
  Time : Scope
      settings: TimeRange=10  YMin=0  YMax=0.5  SaveName=ComputationTime
  wires:
  Bus Selector/1 -> Time/1  "<ComputationTime[s]>"
  [SimCoreInfo] -> Bus Selector/1

== system Demo_3D_Dynamics_cs/VISUWheels_BMW_X5_1 ==
  Wheels : Inport
  Demux : Demux  Outputs=[3 3 3 3 3 3 3 3]
  Saturation{,2,4,6} (4 alike) : Saturate  UpperLimit=[0.2 0.2 0.5]  LowerLimit=[-0.2 -0.2 -0.5]
  Saturation{1,3,5,8} (4 alike) : Saturate  UpperLimit=[30 inf 30]  LowerLimit=[-30 -inf -30]
  conv_RotWheelFL : Subsystem
  conv_RotWheelFR : Subsystem
  conv_RotWheelRL : Subsystem
  conv_RotWheelRR : Subsystem
  conv_TransWheelFL : Subsystem  mask(Translation node configuration){tp=Front-Left Wheel, gains=off, Gain_xISO=1, Gain_yISO=1, Gain_zISO=1}
      mask prompts: tp "Type"; gains "Edit scaling factors?"; Gain_xISO "Scaling factor in x-direction (ISO-convention)"; Gain_yISO "Scaling factor in y-direction (ISO-convention)"; Gain_zISO "Scaling factor in z-direction (ISO-convention)"
      mask init:
      | Visu_ini_param('BMW_X5',tp);
      mask StyleString: popup(Front-Left Wheel|Front-Right Wheel|Rear-Left Wheel|Rear-Right Wheel|Left Seat|Right Seat),checkbox,edit,edit,edit
      mask CallbackString:
      | |if strcmp(get_param(gcb, 'gains'),'on')
      |     set_param(gcb,'MaskVisibilities',{'on','on','on','on','on'})
      | else
      |     set_param(gcb,'MaskVisibilities',{'on','on','off','off','off'})
      | end|||
  conv_TransWheelFR : Subsystem  mask(Translation node configuration){tp=Front-Right Wheel, gains=off, Gain_xISO=1, Gain_yISO=1, Gain_zISO=1}
      mask prompts: tp "Type"; gains "Edit scaling factors?"; Gain_xISO "Scaling factor in x-direction (ISO-convention)"; Gain_yISO "Scaling factor in y-direction (ISO-convention)"; Gain_zISO "Scaling factor in z-direction (ISO-convention)"
      mask init:
      | Visu_ini_param('BMW_X5',tp);
      mask StyleString: popup(Front-Left Wheel|Front-Right Wheel|Rear-Left Wheel|Rear-Right Wheel|Left Seat|Right Seat),checkbox,edit,edit,edit
      mask CallbackString:
      | |if strcmp(get_param(gcb, 'gains'),'on')
      |     set_param(gcb,'MaskVisibilities',{'on','on','on','on','on'})
      | else
      |     set_param(gcb,'MaskVisibilities',{'on','on','off','off','off'})
      | end|||
  conv_TransWheelRL : Subsystem  mask(Translation node configuration){tp=Rear-Left Wheel, gains=off, Gain_xISO=1, Gain_yISO=1, Gain_zISO=1}
      mask prompts: tp "Type"; gains "Edit scaling factors?"; Gain_xISO "Scaling factor in x-direction (ISO-convention)"; Gain_yISO "Scaling factor in y-direction (ISO-convention)"; Gain_zISO "Scaling factor in z-direction (ISO-convention)"
      mask init:
      | Visu_ini_param('BMW_X5',tp);
      mask StyleString: popup(Front-Left Wheel|Front-Right Wheel|Rear-Left Wheel|Rear-Right Wheel|Left Seat|Right Seat),checkbox,edit,edit,edit
      mask CallbackString:
      | |if strcmp(get_param(gcb, 'gains'),'on')
      |     set_param(gcb,'MaskVisibilities',{'on','on','on','on','on'})
      | else
      |     set_param(gcb,'MaskVisibilities',{'on','on','off','off','off'})
      | end|||
  conv_TransWheelRR : Subsystem  mask(Translation node configuration){tp=Rear-Right Wheel, gains=off, Gain_xISO=1, Gain_yISO=1, Gain_zISO=1}
      mask prompts: tp "Type"; gains "Edit scaling factors?"; Gain_xISO "Scaling factor in x-direction (ISO-convention)"; Gain_yISO "Scaling factor in y-direction (ISO-convention)"; Gain_zISO "Scaling factor in z-direction (ISO-convention)"
      mask init:
      | Visu_ini_param('BMW_X5',tp);
      mask StyleString: popup(Front-Left Wheel|Front-Right Wheel|Rear-Left Wheel|Rear-Right Wheel|Left Seat|Right Seat),checkbox,edit,edit,edit
      mask CallbackString:
      | |if strcmp(get_param(gcb, 'gains'),'on')
      |     set_param(gcb,'MaskVisibilities',{'on','on','on','on','on'})
      | else
      |     set_param(gcb,'MaskVisibilities',{'on','on','off','off','off'})
      | end|||
  visu_RotWheelFL : Subsystem  mask(ToSensorWorld){PortName=visu_RotWheelFL_0, PortIndex=18, PortWidth=4, TimeStep=10/200}
      mask prompts: PortName "Port Name [-]"; PortIndex "Index [-]"; PortWidth "Port Dimensions [-]"; TimeStep "Upload Period [s]"
      mask help: Sends signal(s) from Simulink to the Sensor World
      mask Help:
      | Sends signal(s) from Simulink to the Sensor World.
      | 
      | - Port Name [-]: specifies the name of the output terminal of the Simulink block.
      | - Index [-]: specifies the start position in the output vector sent to the Sensor World
      | - Port dimensions [-]: specifies the width (number of scalars) of the output port
      | - Upload period [s]: specifies the upload period (in seconds) of the port.
      mask Display: port_label('input', 1, PortName)
  visu_RotWheelFR : Subsystem  mask(ToSensorWorld){PortName=visu_RotWheelFR_0, PortIndex=25, PortWidth=4, TimeStep=10/200}
      mask prompts: PortName "Port Name [-]"; PortIndex "Index [-]"; PortWidth "Port Dimensions [-]"; TimeStep "Upload Period [s]"
      mask help: Sends signal(s) from Simulink to the Sensor World
      mask Help:
      | Sends signal(s) from Simulink to the Sensor World.
      | 
      | - Port Name [-]: specifies the name of the output terminal of the Simulink block.
      | - Index [-]: specifies the start position in the output vector sent to the Sensor World
      | - Port dimensions [-]: specifies the width (number of scalars) of the output port
      | - Upload period [s]: specifies the upload period (in seconds) of the port.
      mask Display: port_label('input', 1, PortName)
  visu_RotWheelRL : Subsystem  mask(ToSensorWorld){PortName=visu_RotWheelRL_0, PortIndex=32, PortWidth=4, TimeStep=10/200}
      mask prompts: PortName "Port Name [-]"; PortIndex "Index [-]"; PortWidth "Port Dimensions [-]"; TimeStep "Upload Period [s]"
      mask help: Sends signal(s) from Simulink to the Sensor World
      mask Help:
      | Sends signal(s) from Simulink to the Sensor World.
      | 
      | - Port Name [-]: specifies the name of the output terminal of the Simulink block.
      | - Index [-]: specifies the start position in the output vector sent to the Sensor World
      | - Port dimensions [-]: specifies the width (number of scalars) of the output port
      | - Upload period [s]: specifies the upload period (in seconds) of the port.
      mask Display: port_label('input', 1, PortName)
  visu_RotWheelRR : Subsystem  mask(ToSensorWorld){PortName=visu_RotWheelRR_0, PortIndex=39, PortWidth=4, TimeStep=10/200}
      mask prompts: PortName "Port Name [-]"; PortIndex "Index [-]"; PortWidth "Port Dimensions [-]"; TimeStep "Upload Period [s]"
      mask help: Sends signal(s) from Simulink to the Sensor World
      mask Help:
      | Sends signal(s) from Simulink to the Sensor World.
      | 
      | - Port Name [-]: specifies the name of the output terminal of the Simulink block.
      | - Index [-]: specifies the start position in the output vector sent to the Sensor World
      | - Port dimensions [-]: specifies the width (number of scalars) of the output port
      | - Upload period [s]: specifies the upload period (in seconds) of the port.
      mask Display: port_label('input', 1, PortName)
  visu_TransWheelFL : Subsystem  mask(ToSensorWorld){PortName=visu_TransWheelFL_0, PortIndex=15, PortWidth=3, TimeStep=10/200}
      mask prompts: PortName "Port Name [-]"; PortIndex "Index [-]"; PortWidth "Port Dimensions [-]"; TimeStep "Upload Period [s]"
      mask help: Sends signal(s) from Simulink to the Sensor World
      mask Help:
      | Sends signal(s) from Simulink to the Sensor World.
      | 
      | - Port Name [-]: specifies the name of the output terminal of the Simulink block.
      | - Index [-]: specifies the start position in the output vector sent to the Sensor World
      | - Port dimensions [-]: specifies the width (number of scalars) of the output port
      | - Upload period [s]: specifies the upload period (in seconds) of the port.
      mask Display: port_label('input', 1, PortName)
  visu_TransWheelFR : Subsystem  mask(ToSensorWorld){PortName=visu_TransWheelFR_0, PortIndex=22, PortWidth=3, TimeStep=10/200}
      mask prompts: PortName "Port Name [-]"; PortIndex "Index [-]"; PortWidth "Port Dimensions [-]"; TimeStep "Upload Period [s]"
      mask help: Sends signal(s) from Simulink to the Sensor World
      mask Help:
      | Sends signal(s) from Simulink to the Sensor World.
      | 
      | - Port Name [-]: specifies the name of the output terminal of the Simulink block.
      | - Index [-]: specifies the start position in the output vector sent to the Sensor World
      | - Port dimensions [-]: specifies the width (number of scalars) of the output port
      | - Upload period [s]: specifies the upload period (in seconds) of the port.
      mask Display: port_label('input', 1, PortName)
  visu_TransWheelRL : Subsystem  mask(ToSensorWorld){PortName=visu_TransWheelRL_0, PortIndex=29, PortWidth=3, TimeStep=10/200}
      mask prompts: PortName "Port Name [-]"; PortIndex "Index [-]"; PortWidth "Port Dimensions [-]"; TimeStep "Upload Period [s]"
      mask help: Sends signal(s) from Simulink to the Sensor World
      mask Help:
      | Sends signal(s) from Simulink to the Sensor World.
      | 
      | - Port Name [-]: specifies the name of the output terminal of the Simulink block.
      | - Index [-]: specifies the start position in the output vector sent to the Sensor World
      | - Port dimensions [-]: specifies the width (number of scalars) of the output port
      | - Upload period [s]: specifies the upload period (in seconds) of the port.
      mask Display: port_label('input', 1, PortName)
  visu_TransWheelRR : Subsystem  mask(ToSensorWorld){PortName=visu_TransWheelRR_0, PortIndex=36, PortWidth=3, TimeStep=10/200}
      mask prompts: PortName "Port Name [-]"; PortIndex "Index [-]"; PortWidth "Port Dimensions [-]"; TimeStep "Upload Period [s]"
      mask help: Sends signal(s) from Simulink to the Sensor World
      mask Help:
      | Sends signal(s) from Simulink to the Sensor World.
      | 
      | - Port Name [-]: specifies the name of the output terminal of the Simulink block.
      | - Index [-]: specifies the start position in the output vector sent to the Sensor World
      | - Port dimensions [-]: specifies the width (number of scalars) of the output port
      | - Upload period [s]: specifies the upload period (in seconds) of the port.
      mask Display: port_label('input', 1, PortName)
  wires:
  conv_RotWheelRR/1(QuaternionVisu [rad]) -> visu_RotWheelRR/1(Y)
  conv_TransWheelRR/1(transVisu [m]) -> visu_TransWheelRR/1(Y)
  conv_RotWheelRL/1(QuaternionVisu [rad]) -> visu_RotWheelRL/1(Y)
  conv_TransWheelRL/1(transVisu [m]) -> visu_TransWheelRL/1(Y)
  conv_RotWheelFR/1(QuaternionVisu [rad]) -> visu_RotWheelFR/1(Y)
  conv_TransWheelFR/1(transVisu [m]) -> visu_TransWheelFR/1(Y)
  conv_RotWheelFL/1(QuaternionVisu [rad]) -> visu_RotWheelFL/1(Y)
  conv_TransWheelFL/1(transVisu [m]) -> visu_TransWheelFL/1(Y)
  Demux/8 -> Saturation5/1
  Demux/7 -> Saturation6/1
  Demux/6 -> Saturation3/1
  Demux/5 -> Saturation4/1
  Demux/4 -> Saturation1/1
  Demux/3 -> Saturation2/1
  Demux/2 -> Saturation8/1
  Demux/1 -> Saturation/1
  Saturation5/1 -> conv_RotWheelRR/1(BryantISO [deg])
  Saturation6/1 -> conv_TransWheelRR/1(transISO [m])
  Saturation3/1 -> conv_RotWheelRL/1(BryantISO [deg])
  Saturation4/1 -> conv_TransWheelRL/1(transISO [m])
  Saturation1/1 -> conv_RotWheelFR/1(BryantISO [deg])
  Saturation2/1 -> conv_TransWheelFR/1(transISO [m])
  Saturation8/1 -> conv_RotWheelFL/1(BryantISO [deg])
  Saturation/1 -> conv_TransWheelFL/1(transISO [m])
  Wheels/1 -> Demux/1  "wheels"

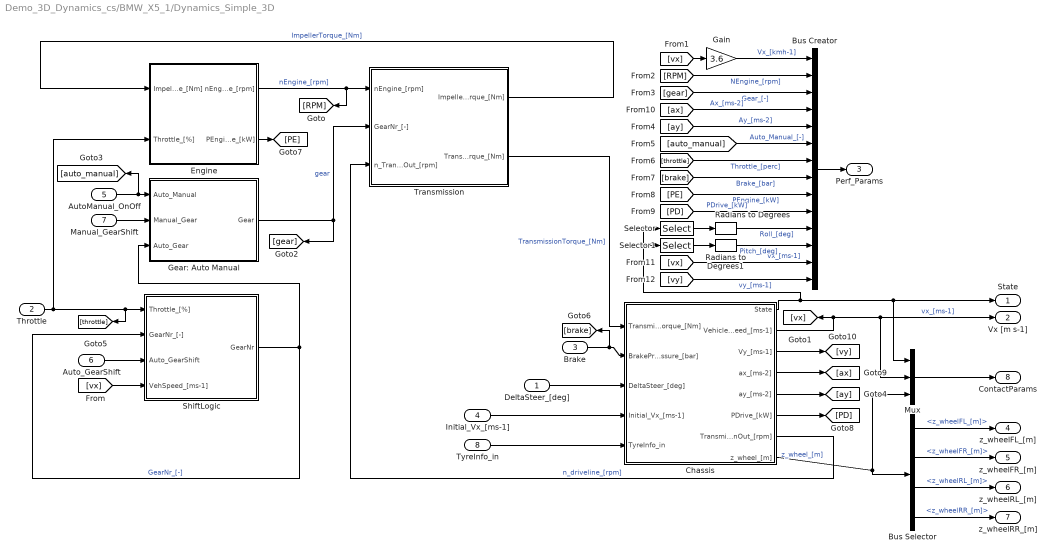
== system Demo_3D_Dynamics_cs/BMW_X5_1/Dynamics_Simple_3D ==
  DeltaSteer_[deg] : Inport
  Throttle : Inport  Port=2
  Brake : Inport  Port=3
  Initial_Vx_[ms-1] : Inport  Port=4
  AutoManual_OnOff : Inport  Port=5
  Auto_GearShift : Inport  Port=6
  Manual_GearShift : Inport  Port=7
  TyreInfo_in : Inport  Port=8
  Bus Creator : BusCreator  Inputs=14
  Bus Selector : BusSelector  OutputSignals=z_wheelFL_[m],z_wheelFR_[m],z_wheelRL_[m],z_wheelRR_[m]
  Chassis : Subsystem
      mask Display: image(imread('Chassis.png'));
  Engine : Subsystem
      mask Display: image(imread('Engine.png'));
  Gain : Gain  Gain=3.6
  Gear: Auto Manual : Subsystem
  Mux : Mux  Inputs=3
  Radians to Degrees : simulink_extras/Transformations/Radians to Degrees  SystemSampleTime=-1
  Radians to Degrees1 : simulink_extras/Transformations/Radians to Degrees  SystemSampleTime=-1
  Selector : Selector  InputPortWidth=9  IndexOptions=Index vector (dialog)  Indices=7  OutputSizes=1
  Selector1 : Selector  InputPortWidth=9  IndexOptions=Index vector (dialog)  Indices=8  OutputSizes=1
  ShiftLogic : Subsystem
      mask Display: image(imread('Gearshift.png'));
  Transmission : Subsystem
      mask Display: image(imread('Transmission.png'));
  State : Outport
  Vx [m s-1] : Outport  Port=2
  Perf_Params : Outport  Port=3
  z_wheelFL_[m] : Outport  Port=4
  z_wheelFR_[m] : Outport  Port=5
  z_wheelRL_[m] : Outport  Port=6
  z_wheelRR_[m] : Outport  Port=7
  ContactParams : Outport  Port=8
  wires:
  Mux/1 -> ContactParams/1
  Bus Selector/4 -> z_wheelRR_[m]/1  "<z_wheelRR_[m]>"
  Bus Selector/3 -> z_wheelRL_[m]/1  "<z_wheelRL_[m]>"
  Bus Selector/2 -> z_wheelFR_[m]/1  "<z_wheelFR_[m]>"
  Bus Selector/1 -> z_wheelFL_[m]/1  "<z_wheelFL_[m]>"
  Chassis/8(z_wheel_[m]) -> Mux/3, Bus Selector/1  "z_wheel_[m]"
  [vy] -> Bus Creator/14  "vy_[ms-1]"
  [vx] -> Bus Creator/13  "vx_[ms-1]"
  Chassis/3(Vy_[ms-1]) -> [vy]
  Chassis/4(ax_[ms-2]) -> [ax]
  Chassis/5(ay_[ms-2]) -> [ay]
  Chassis/6(PDrive_[kW]) -> [PD]
  Brake/1 -> [brake], Chassis/2(BrakePressure_[bar])
  TyreInfo_in/1 -> Chassis/5(TyreInfo_in)
  [vx] -> ShiftLogic/4(VehSpeed_[ms-1])
  Gear: Auto Manual/1(Gear) -> Transmission/2(GearNr_[-]), [gear]  "gear"
  Manual_GearShift/1 -> Gear: Auto Manual/2(Manual_Gear)
  AutoManual_OnOff/1 -> Gear: Auto Manual/1(Auto_Manual), [auto_manual]
  Chassis/2(VehicleSpeed_[ms-1]) -> Mux/2, Vx [m s-1]/1, [vx]  "vx_[ms-1]"
  Chassis/7(TransmissionOut_[rpm]) -> Transmission/3(n_TransmissionOut_[rpm])  "n_driveline_[rpm]"
  Auto_GearShift/1 -> ShiftLogic/3(Auto_GearShift)
  Throttle/1 -> Engine/2(Throttle_[%]), ShiftLogic/1(Throttle_[%]), [throttle]
  Initial_Vx_[ms-1]/1 -> Chassis/4(Initial_Vx_[ms-1])
  DeltaSteer_[deg]/1 -> Chassis/3(DeltaSteer_[deg])
  Chassis/1(State) -> Mux/1, State/1, Selector/1, Selector1/1
  Engine/1(nEngine_[rpm]) -> [RPM], Transmission/1(nEngine_[rpm])  "nEngine_[rpm]"
  ShiftLogic/1(GearNr) -> Gear: Auto Manual/3(Auto_Gear), ShiftLogic/2(GearNr_[-])  "GearNr_[-]"
  Transmission/2(TransmissionTorque_[Nm]) -> Chassis/1(TransmissionTorque_[Nm])  "TransmissionTorque_[Nm]"
  Transmission/1(ImpellerTorque_[Nm]) -> Engine/1(ImpellerTorque_[Nm])  "ImpellerTorque_[Nm]"
  Gain/1 -> Bus Creator/1  "Vx_[kmh-1]"
  [RPM] -> Bus Creator/2  "NEngine_[rpm]"
  [gear] -> Bus Creator/3  "Gear_[-]"
  [ay] -> Bus Creator/5  "Ay_[ms-2]"
  [auto_manual] -> Bus Creator/6  "Auto_Manual_[-]"
  [throttle] -> Bus Creator/7  "Throttle_[perc]"
  [brake] -> Bus Creator/8  "Brake_[bar]"
  Engine/2(PEngine_[kW]) -> [PE]
  Bus Creator/1 -> Perf_Params/1
  [PE] -> Bus Creator/9  "PEngine_[kW]"
  Radians to Degrees/1 -> Bus Creator/11  "Roll_[deg]"
  Radians to Degrees1/1 -> Bus Creator/12  "Pitch_[deg]"
  [PD] -> Bus Creator/10  "PDrive_[kW]"
  Selector/1 -> Radians to Degrees/1
  Selector1/1 -> Radians to Degrees1/1
  [vx] -> Gain/1
  [ax] -> Bus Creator/4  "Ax_[ms-2]"

== system Demo_3D_Dynamics_cs/BMW_X5_1/PathFollower_1 ==
  TrajOffset_x,y,Y [m,m,deg] : Inport
  ActorOffset_Left(+) / Right(-) [m] : Inport  Port=2
  position x,y,Y [m,m,deg] : Inport  Port=3
  Initial Velocity [m/s] : Inport  Port=4
  Desired Velocity [m/s] : Inport  Port=5
  velocity [m/s] : Inport  Port=6
  CTRL REFERENCES : Subsystem
  Calculate shifted p0 wrt COG : Subsystem
  DELTA CTRL : Subsystem
  Demux : Demux  Outputs=3
  Gain : Gain  Gain=1*pi/180
  Goto Tag Visibility : GotoTagVisibility  GotoTag=PreviewDistance
  Goto Tag Visibility1 : GotoTagVisibility  GotoTag=v_actual
  Memory1 : Memory
  Memory2 : Memory
  Memory3 : Memory
  Mux : Mux  Inputs=3
  Preview distance  velocity dependent : Lookup  InputValues=[0 20 30 40 50 60 70 80 90 100 120]  Table=[1 1 2 3 4 5 6 7 10 13.33 20]
  THROTTLE CTRL : Subsystem
  sign1 : Gain  Gain=3.6
  delta_steerwheel [deg] : Outport
  throttle [%] : Outport  Port=2
  brake pressure [bar] : Outport  Port=3
  v0 [m/s] : Outport  Port=4
  Auto_GearShift : Outport  Port=5
  Actor/Traj_distance [m] : Outport  Port=6
  Actor/Traj_angle [deg] : Outport  Port=7
  tag scope: PreviewDistance=scoped, v_actual=scoped
  wires:
  Memory3/1 -> CTRL REFERENCES/4(ActorOffset_Left(+) / Right(-)_[m])
  THROTTLE CTRL/4(Auto_GearShift) -> Auto_GearShift/1
  THROTTLE CTRL/2(brake pressure [bar]) -> brake pressure [bar]/1
  Memory2/1 -> THROTTLE CTRL/1(v_actual [m/s]), [v_actual]
  Memory1/1 -> DELTA CTRL/1(p0), CTRL REFERENCES/1(Pos x,y,Y [m,m,rad])
  sign1/1 -> Preview distance  velocity dependent/1
  Initial Velocity [m/s]/1 -> THROTTLE CTRL/3(Initial Velocity [m/s])
  velocity [m/s]/1 -> Memory2/1
  CTRL REFERENCES/1(pvp  [m,m]) -> DELTA CTRL/2(pvp)
  CTRL REFERENCES/2(pref_pvp [m,m]) -> DELTA CTRL/3(pref_pvp)
  Gain/1 -> Mux/3
  DELTA CTRL/1(delta_steerwheel [deg]) -> delta_steerwheel [deg]/1
  Mux/1 -> CTRL REFERENCES/3(TrajOffset [m,m,rad])
  CTRL REFERENCES/3(pref_0 [m,m]) -> DELTA CTRL/4(pref0)
  THROTTLE CTRL/3(v0 [m/s]) -> v0 [m/s]/1
  THROTTLE CTRL/1(throttle [%]) -> throttle [%]/1
  [v_actual] -> sign1/1
  Preview distance  velocity dependent/1 -> [PreviewDistance], CTRL REFERENCES/2(Position Preview Distance [m])
  Desired Velocity [m/s]/1 -> THROTTLE CTRL/2(Desired Velocity [m/s])
  ActorOffset_Left(+) / Right(-) [m]/1 -> Memory3/1
  Demux/1 -> Mux/1
  Demux/2 -> Mux/2
  Demux/3 -> Gain/1
  TrajOffset_x,y,Y [m,m,deg]/1 -> Demux/1
  Calculate shifted p0 wrt COG/1(position x,y,Y [m,m,rad]) -> Memory1/1
  position x,y,Y [m,m,deg]/1 -> Calculate shifted p0 wrt COG/1(position x,y,Y [m,m,deg])
  CTRL REFERENCES/4(Actor/Traj_distance [m]) -> Actor/Traj_distance [m]/1
  CTRL REFERENCES/5(Actor/Traj_angle [deg]) -> Actor/Traj_angle [deg]/1

== system Demo_3D_Dynamics_cs/BMW_X5_1/PreScan_Contact_Sensor ==
  ContactParams : Inport  SampleTime=TimeStep
  Steer Angle Front [deg] : Inport  Port=2
  Steer Angle Rear [deg] : Inport  Port=3
  Bus Creator2 : BusCreator
  Demux : Demux
  Demux1 : Demux  Outputs=[9 1 4]
  Demux2 : Demux
  Level-2 MATLAB S-Function : M-S-Function  FunctionName=msfcn_wheelContacts  Parameters=NumberOfWheels, MaxContactPoints, WheelRadius, WheelWidth  mask{NumberOfWheels=4, MaxContactPoints=4, WheelRadius=[wheelRadius wheelRadius wheelRadius wheelRadius], WheelWidth=0.2}
      mask prompts: NumberOfWheels "Number of Wheels:"; MaxContactPoints "Maximum number of Contact Points:"; WheelRadius "Wheel Radius:"; WheelWidth "Wheel Width:"
      mask Display: disp('Contact Sensor')
  Level-2 MATLAB S-Function1 : M-S-Function  FunctionName=msfcn_CollisionConv  Parameters=NumberOfWheels hcog b  mask{NumberOfWheels=4}
      mask prompts: NumberOfWheels "Number of Wheels:"
      settings: AttributesFormatString=Wheels = %<NumberOfWheels>
      mask Display:
      | port_label('input', 1,'Vehicle wrt World')
      | port_label('input', 2,'Wheels wrt World')
  Mux6 : Mux  Inputs=2
  Tire Collision Demux : Subsystem
  Tire Collision Demux1 : Subsystem
  Tire Collision Demux2 : Subsystem
  Tire Collision Demux3 : Subsystem
  Vehicle Local to World : Subsystem
  Wheels Local to World : Subsystem  Tag=MuxWheels
      settings: DeleteFcn=PreScanBlockDeleteFcn;
      mask Type: PreScan Mux Block:
  Results : Outport
  wires:
  Demux1/3 -> Demux2/1
  Demux1/1 -> Vehicle Local to World/1(State)
  ContactParams/1 -> Demux1/1
  Bus Creator2/1 -> Results/1
  Steer Angle Rear [deg]/1 -> Wheels Local to World/2(Steer Angle Rear [deg])
  Steer Angle Front [deg]/1 -> Wheels Local to World/1(Steer Angle Front [deg])
  Demux2/4 -> Wheels Local to World/7(zDisp RR [m])
  Demux2/3 -> Wheels Local to World/6(zDisp RL [m])
  Demux2/2 -> Wheels Local to World/5(zDisp FR [m])
  Demux2/1 -> Wheels Local to World/4(zDisp FL [m])
  Demux1/2 -> Wheels Local to World/3(Velocity [m/s])
  Wheels Local to World/1(Wheel Poses) -> Level-2 MATLAB S-Function1/2
  Vehicle Local to World/2(Orientation) -> Mux6/2
  Vehicle Local to World/1(Position) -> Mux6/1
  Tire Collision Demux3/1(bus out) -> Bus Creator2/4  "TireRR"
  Tire Collision Demux2/1(bus out) -> Bus Creator2/3  "TireRL"
  Tire Collision Demux1/1(bus out) -> Bus Creator2/2  "TireFR"
  Tire Collision Demux/1(bus out) -> Bus Creator2/1  "TireFL"
  Demux/4 -> Tire Collision Demux3/1(demux in)
  Demux/3 -> Tire Collision Demux2/1(demux in)
  Demux/2 -> Tire Collision Demux1/1(demux in)
  Demux/1 -> Tire Collision Demux/1(demux in)
  Level-2 MATLAB S-Function/1 -> Demux/1
  Level-2 MATLAB S-Function1/1 -> Level-2 MATLAB S-Function/1
  Mux6/1 -> Level-2 MATLAB S-Function1/1

== system Demo_3D_Dynamics_cs/BMW_X5_1/SELF_Demux ==
  SELF : Inport
  Demux1 : Demux  Outputs=3
  Demux2 : Demux  Outputs=3
  Demux3 : Demux  Outputs=[3 3 1 1]
  Demux4 : Demux  Outputs=3
  Gain : Gain  Gain=180/pi
  Gain1 : Gain  Gain=180/pi
  Selector : Selector  InputPortWidth=3  IndexOptions=Index vector (dialog)  Indices=[3]  OutputSizes=1
  compas converter : Subsystem
  xyz2GPS : PreScanUsefulBlocks/xyz2GPS  CoordinateCount=1  GPS_base=[0.000000 0.000000 0.000]
  x [m] : Outport
  y [m] : Outport  Port=2
  z [m] : Outport  Port=3
  rotx [deg] : Outport  Port=4
  roty [deg] : Outport  Port=5
  rotz [deg] : Outport  Port=6
  GPS lat [deg] : Outport  Port=7
  GPS long [deg] : Outport  Port=8
  GPS alt [m] : Outport  Port=9
  velocity [m/s] : Outport  Port=10
  heading [deg] : Outport  Port=11
  yaw rate [deg/s] : Outport  Port=12
  wires:
  Demux3/4 -> Gain1/1
  Gain1/1 -> yaw rate [deg/s]/1
  Demux3/3 -> velocity [m/s]/1
  compas converter/1(heading [deg]) -> heading [deg]/1
  xyz2GPS/1 -> Demux4/1
  Demux4/3 -> GPS alt [m]/1
  Demux4/2 -> GPS long [deg]/1
  Demux4/1 -> GPS lat [deg]/1
  Demux3/2 -> Gain/1, Selector/1
  Demux3/1 -> xyz2GPS/1, Demux1/1
  SELF/1 -> Demux3/1
  Demux2/3 -> rotz [deg]/1
  Demux2/2 -> roty [deg]/1
  Demux2/1 -> rotx [deg]/1
  Demux1/3 -> z [m]/1
  Demux1/2 -> y [m]/1
  Demux1/1 -> x [m]/1
  Gain/1 -> Demux2/1
  Selector/1 -> compas converter/1(rotz [rad])

== system Demo_3D_Dynamics_cs/BMW_X5_1/Trajectories ==
  Traj2State1 : Subsystem  Tag=Traj2State
      settings: DeleteFcn=PreScanBlockDeleteFcn;
      mask Type: PreScan Demux Block:
  Trajectory_1 : Subsystem  Tag=Trajectory  mask(PreScan Source Block: Trajectory){FileName='Trajectory_1.mat', TimeStep=10/200}
      mask prompts: TimeStep "Time Step [s]"
      mask help:
      | The Trajectory block contains the trajectories defined in the PreScan Experiment Editor. The output of the trajectory block is the (vehicle) State.
      |
      | For more information, please click Help.
      mask init:
      | [direc,name]=fileparts(get_param(bdroot, 'FileName'));
      | load([direc,'/Trajectories/',FileName])
      | trajectory=trajectory';
      | 
      | traj.time=trajectory(:,1);%[];
      | traj.signals.values=trajectory(:,2:19);
      | traj.dimensions=18;
      | traj.label='';
      | 
      | SampleTime=traj.time(2)-traj.time(1);
      settings: DeleteFcn=PreScanBlockDeleteFcn;
      mask Help: eval('openHelp(312)')
      mask Display: fprintf(FileName)
  Trajectory_1_Offset : Constant  Tag=TrajectoryOffset  Value="[0  0  0  0  0  0]"
  State : Outport  Tag=TrajOutport
  wires:
  Trajectory_1/1(trajectory) -> Traj2State1/1(Traj Org)
  Trajectory_1_Offset/1 -> Traj2State1/2(Offset)
  Traj2State1/1(state) -> State/1

== system Demo_3D_Dynamics_cs/BMW_X5_1/VISUWheels_Mux ==
  Steer Angle Front [deg] : Inport  SampleTime=TimeStep
  Steer Angle Rear [deg] : Inport  Port=2  SampleTime=TimeStep
  Velocity [m/s] : Inport  Port=3  SampleTime=TimeStep
  zDisp FL [m] : Inport  Port=4  SampleTime=TimeStep
  zDisp FR [m] : Inport  Port=5  SampleTime=TimeStep
  zDisp RL [m] : Inport  Port=6  SampleTime=TimeStep
  zDisp RR [m] : Inport  Port=7  SampleTime=TimeStep
  Constant{,1..3} (4 alike) : Constant  Value=[0 0]  SampleTime=TimeStep
  Constant{4..7} (4 alike) : Constant  Value=0  SampleTime=TimeStep
  Discrete-Time Integrator : DiscreteIntegrator  SampleTime=TimeStep  ICPrevOutput=DiscIntNeverNeededParam  ICPrevScaledInput=DiscIntNeverNeededParam
  Mux{,1..3} (4 alike) : Mux  Inputs=3
  Mux{4,6..8} (4 alike) : Mux  Inputs=[2 1]
  Mux5 : Mux  Inputs=[3 3 3 3 3 3 3 3]
  Radians to Degrees : simulink_extras/Transformations/Radians to Degrees  SystemSampleTime=-1
  omega=V/Rwheel : Gain  Gain=1/0.29
  Wheels : Outport
  wires:
  Mux7/1 -> Mux5/5  "xyz displacement RL [m]"
  Discrete-Time Integrator/1 -> Mux/2, Mux1/2, Mux2/2, Mux3/2  "roty"
  Radians to Degrees/1 -> Discrete-Time Integrator/1
  Constant7/1 -> Mux3/1  "rotx"
  Constant6/1 -> Mux2/1  "rotx"
  Constant5/1 -> Mux1/1  "rotx"
  Constant4/1 -> Mux/1  "rotx"
  Steer Angle Front [deg]/1 -> Mux1/3, Mux/3  "rotz"
  Steer Angle Rear [deg]/1 -> Mux3/3, Mux2/3  "rotz"
  Mux8/1 -> Mux5/7  "xyz displacement RR [m]"
  Mux6/1 -> Mux5/3  "xyz displacement FR [m]"
  Mux4/1 -> Mux5/1  "xyz displacement FL [m]"
  Constant3/1 -> Mux8/1
  Constant2/1 -> Mux7/1
  Constant1/1 -> Mux6/1
  Constant/1 -> Mux4/1
  zDisp RR [m]/1 -> Mux8/2
  zDisp RL [m]/1 -> Mux7/2
  zDisp FR [m]/1 -> Mux6/2
  zDisp FL [m]/1 -> Mux4/2
  Mux5/1 -> Wheels/1
  omega=V/Rwheel/1 -> Radians to Degrees/1  "rotational speed [rad/s]"
  Velocity [m/s]/1 -> omega=V/Rwheel/1
  Mux1/1 -> Mux5/4  "xyz rotation FR [deg]"
  Mux/1 -> Mux5/2  "xyz rotation FL [deg]"
  Mux3/1 -> Mux5/8  "xyz rotation RR [deg]"
  Mux2/1 -> Mux5/6  "xyz rotation RL [deg]"

== system Demo_3D_Dynamics_cs/STATE_BMW_X5_1/Acceleration ==
  Y : Inport
  Assignment : Assignment  IndexMode=Zero-based  SampleTime=TimeStep  IndexOptions=Starting index (dialog)  Indices=PortIndex  OutputSizes=[1 1]
  Data Store Read : DataStoreRead  DataStoreName=SimCoreActuators  SampleTime=TimeStep
  Data Store Write : DataStoreWrite  DataStoreName=SimCoreActuators
  wires:
  Assignment/1 -> Data Store Write/1
  Data Store Read/1 -> Assignment/1
  Y/1 -> Assignment/2

== system Demo_3D_Dynamics_cs/STATE_BMW_X5_1/Position ==
  Y : Inport
  Assignment : Assignment  IndexMode=Zero-based  SampleTime=TimeStep  IndexOptions=Starting index (dialog)  Indices=PortIndex  OutputSizes=[1 1]
  Data Store Read : DataStoreRead  DataStoreName=SimCoreActuators  SampleTime=TimeStep
  Data Store Write : DataStoreWrite  DataStoreName=SimCoreActuators
  wires:
  Y/1 -> Assignment/2
  Data Store Read/1 -> Assignment/1
  Assignment/1 -> Data Store Write/1

== system Demo_3D_Dynamics_cs/STATE_BMW_X5_1/RPY ==
  Y : Inport
  Assignment : Assignment  IndexMode=Zero-based  SampleTime=TimeStep  IndexOptions=Starting index (dialog)  Indices=PortIndex  OutputSizes=[1 1]
  Data Store Read : DataStoreRead  DataStoreName=SimCoreActuators  SampleTime=TimeStep
  Data Store Write : DataStoreWrite  DataStoreName=SimCoreActuators
  wires:
  Assignment/1 -> Data Store Write/1
  Data Store Read/1 -> Assignment/1
  Y/1 -> Assignment/2

== system Demo_3D_Dynamics_cs/STATE_BMW_X5_1/Velocity ==
  Y : Inport
  Assignment : Assignment  IndexMode=Zero-based  SampleTime=TimeStep  IndexOptions=Starting index (dialog)  Indices=PortIndex  OutputSizes=[1 1]
  Data Store Read : DataStoreRead  DataStoreName=SimCoreActuators  SampleTime=TimeStep
  Data Store Write : DataStoreWrite  DataStoreName=SimCoreActuators
  wires:
  Assignment/1 -> Data Store Write/1
  Data Store Read/1 -> Assignment/1
  Y/1 -> Assignment/2

== system Demo_3D_Dynamics_cs/STATE_BMW_X5_1/velRPY ==
  Y : Inport
  Assignment : Assignment  IndexMode=Zero-based  SampleTime=TimeStep  IndexOptions=Starting index (dialog)  Indices=PortIndex  OutputSizes=[1 1]
  Data Store Read : DataStoreRead  DataStoreName=SimCoreActuators  SampleTime=TimeStep
  Data Store Write : DataStoreWrite  DataStoreName=SimCoreActuators
  wires:
  Assignment/1 -> Data Store Write/1
  Data Store Read/1 -> Assignment/1
  Y/1 -> Assignment/2
